simulink library "AERO_lib"  (R2015a)
settings: Solver=ode45  StartTime=0.0  StopTime=10.0  RelTol=1e-3
values from neighbouring files (symbols this model uses):
  VAF = {}    [setup_aero.m]
libraries: simulink x8
settings Model: Creator=Andrew  LastModifiedBy=Andrew

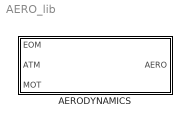
== system AERO_lib ==
  AERODYNAMICS : Subsystem

== system AERO_lib/AERODYNAMICS ==
  EOM : Inport
  ATM : Inport  Port=2
  MOT : Inport  Port=3
  AERODYNAMIC PROPERTIES : Subsystem
  Bus Creator : BusCreator  Inputs=6
  Bus Selector : BusSelector  OutputSignals=SONIC_VEL,TEMP,RHO
  Bus Selector1 : BusSelector  OutputSignals=signal1,signal2
  Bus Selector2 : BusSelector  OutputSignals=signal1,signal2
  AERO : Outport
  wires:
  Bus Selector2/2 -> AERODYNAMIC PROPERTIES/8(MOTOR DIAMETER)  "<signal2>"
  Bus Selector2/1 -> AERODYNAMIC PROPERTIES/7(THRUST ACTIVE)  "<signal1>"
  Bus Selector/3 -> AERODYNAMIC PROPERTIES/6(RHO)  "<RHO>"
  Bus Selector/2 -> AERODYNAMIC PROPERTIES/5(TEMP)  "<TEMP>"
  Bus Selector/1 -> AERODYNAMIC PROPERTIES/4(a (m/s))  "<SONIC_VEL>"
  AERODYNAMIC PROPERTIES/1(X_CP_TOT) -> Bus Creator/1  "X_CP"
  AERODYNAMIC PROPERTIES/2(X_CP_FIN) -> Bus Creator/2  "FIN_CP"
  AERODYNAMIC PROPERTIES/3(Reynolds Number) -> Bus Creator/3  "Re"
  AERODYNAMIC PROPERTIES/4(Cm_Damp) -> Bus Creator/4  "CM_DAMP"
  AERODYNAMIC PROPERTIES/5(CD_TOTAL) -> Bus Creator/5  "CD_TOT"
  AERODYNAMIC PROPERTIES/6(CD_ALL) -> Bus Creator/6  "CD_ALL"
  Bus Creator/1 -> AERO/1
  ATM/1 -> Bus Selector/1
  EOM/1 -> Bus Selector1/1
  MOT/1 -> Bus Selector2/1

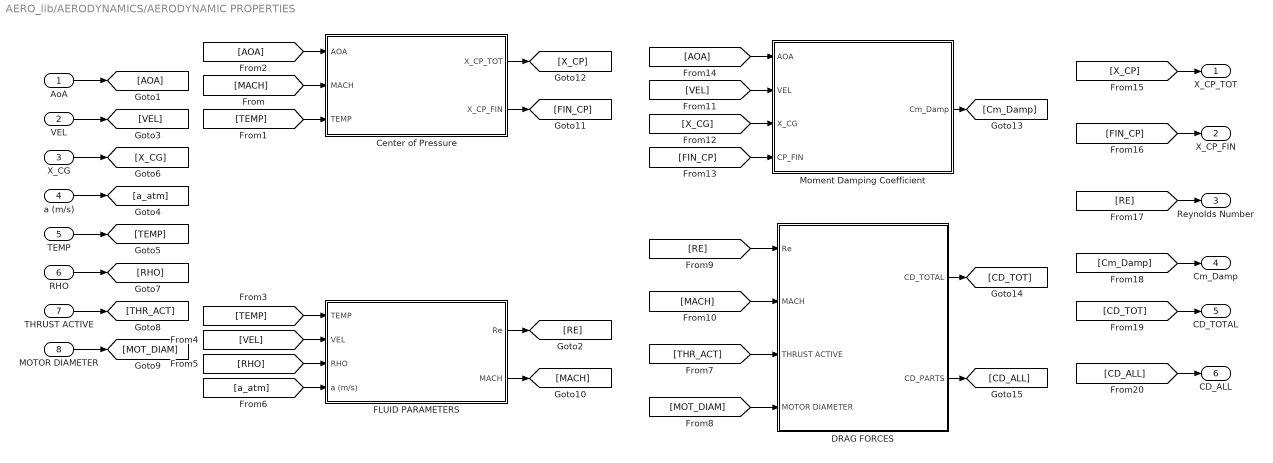
== system AERO_lib/AERODYNAMICS/AERODYNAMIC PROPERTIES ==
  AoA : Inport
  VEL : Inport  Port=2
  X_CG : Inport  Port=3
  a (m/s) : Inport  Port=4
  TEMP : Inport  Port=5
  RHO : Inport  Port=6
  THRUST ACTIVE : Inport  Port=7
  MOTOR DIAMETER : Inport  Port=8
  Center of Pressure : Subsystem
  DRAG FORCES : Subsystem
  FLUID PARAMETERS : Subsystem
  Moment Damping Coefficient : Subsystem
  X_CP_TOT : Outport
  X_CP_FIN : Outport  Port=2
  Reynolds Number : Outport  Port=3
  Cm_Damp : Outport  Port=4
  CD_TOTAL : Outport  Port=5
  CD_ALL : Outport  Port=6
  wires:
  a (m/s)/1 -> [a_atm]
  AoA/1 -> [AOA]
  VEL/1 -> [VEL]
  TEMP/1 -> [TEMP]
  X_CG/1 -> [X_CG]
  RHO/1 -> [RHO]
  THRUST ACTIVE/1 -> [THR_ACT]
  MOTOR DIAMETER/1 -> [MOT_DIAM]
  [MACH] -> Center of Pressure/2(MACH)
  [TEMP] -> Center of Pressure/3(TEMP)
  [AOA] -> Center of Pressure/1(AOA)
  [TEMP] -> FLUID PARAMETERS/1(TEMP)
  [RHO] -> FLUID PARAMETERS/3(RHO)
  [a_atm] -> FLUID PARAMETERS/4(a (m/s))
  [VEL] -> FLUID PARAMETERS/2(VEL)
  [THR_ACT] -> DRAG FORCES/3(THRUST ACTIVE)
  [MOT_DIAM] -> DRAG FORCES/4(MOTOR DIAMETER)
  [MACH] -> DRAG FORCES/2(MACH)
  [RE] -> DRAG FORCES/1(Re)
  FLUID PARAMETERS/1(Re) -> [RE]
  FLUID PARAMETERS/2(MACH) -> [MACH]
  Center of Pressure/1(X_CP_TOT) -> [X_CP]
  Center of Pressure/2(X_CP_FIN) -> [FIN_CP]
  [AOA] -> Moment Damping Coefficient/1(AOA)
  [VEL] -> Moment Damping Coefficient/2(VEL)
  [X_CG] -> Moment Damping Coefficient/3(X_CG)
  [FIN_CP] -> Moment Damping Coefficient/4(CP_FIN)
  DRAG FORCES/1(CD_TOTAL) -> [CD_TOT]
  DRAG FORCES/2(CD_PARTS) -> [CD_ALL]
  Moment Damping Coefficient/1(Cm_Damp) -> [Cm_Damp]
  [X_CP] -> X_CP_TOT/1
  [FIN_CP] -> X_CP_FIN/1
  [RE] -> Reynolds Number/1
  [Cm_Damp] -> Cm_Damp/1
  [CD_TOT] -> CD_TOTAL/1
  [CD_ALL] -> CD_ALL/1

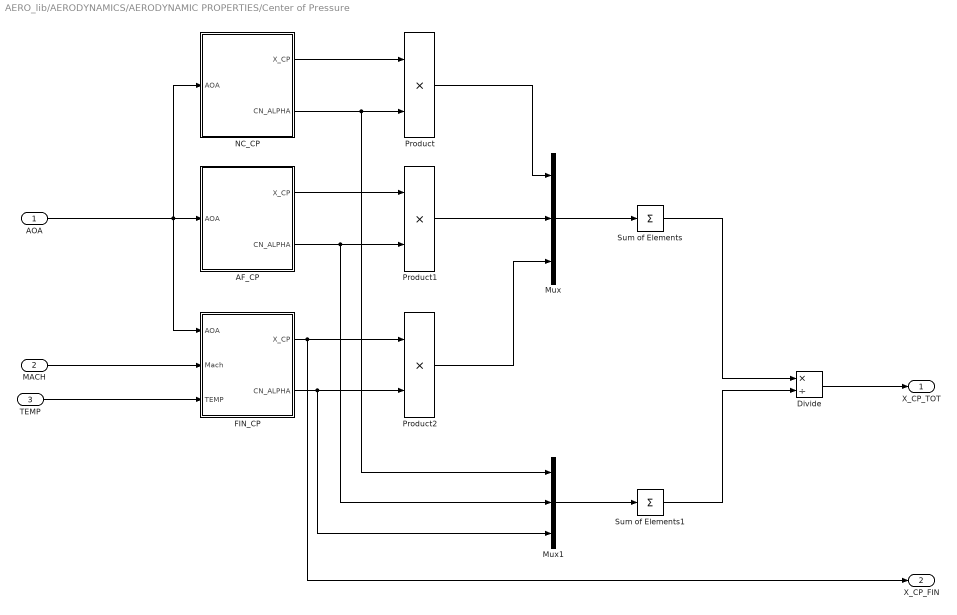
== system AERO_lib/AERODYNAMICS/AERODYNAMIC PROPERTIES/Center of Pressure ==
  AOA : Inport
  MACH : Inport  Port=2
  TEMP : Inport  Port=3
  AF_CP : Subsystem
  Divide : Product  Inputs=*/
  FIN_CP : Subsystem
  Mux : Mux  Inputs=3
  Mux1 : Mux  Inputs=3
  NC_CP : Subsystem
  Product : Product
  Product1 : Product
  Product2 : Product
  Sum of Elements : Sum  Inputs=+
  Sum of Elements1 : Sum  Inputs=+
  X_CP_TOT : Outport
  X_CP_FIN : Outport  Port=2
  wires:
  AOA/1 -> FIN_CP/1(AOA), NC_CP/1(AOA), AF_CP/1(AOA)
  MACH/1 -> FIN_CP/2(Mach)
  NC_CP/1(X_CP) -> Product/1
  AF_CP/2(CN_ALPHA) -> Mux1/2, Product1/2
  Product1/1 -> Mux/2
  Divide/1 -> X_CP_TOT/1
  Sum of Elements/1 -> Divide/1
  Product/1 -> Mux/1
  Mux1/1 -> Sum of Elements1/1
  AF_CP/1(X_CP) -> Product1/1
  NC_CP/2(CN_ALPHA) -> Mux1/1, Product/2
  Mux/1 -> Sum of Elements/1
  Sum of Elements1/1 -> Divide/2
  FIN_CP/1(X_CP) -> X_CP_FIN/1, Product2/1
  Product2/1 -> Mux/3
  FIN_CP/2(CN_ALPHA) -> Product2/2, Mux1/3
  TEMP/1 -> FIN_CP/3(TEMP)

== system AERO_lib/AERODYNAMICS/AERODYNAMIC PROPERTIES/DRAG FORCES ==
  Re : Inport
  MACH : Inport  Port=2
  THRUST ACTIVE : Inport  Port=3
  MOTOR DIAMETER : Inport  Port=4
  Add : Sum
  Body Drag : Subsystem
  Mux : Mux  Inputs=2
  Skin Friction Drag : Subsystem
  CD_TOTAL : Outport
  CD_PARTS : Outport  Port=2
  wires:
  MACH/1 -> Body Drag/1(MACH), Skin Friction Drag/2(MACH)
  Re/1 -> Skin Friction Drag/1(Re)
  MOTOR DIAMETER/1 -> Body Drag/3(MOTOR DIAMETER)
  THRUST ACTIVE/1 -> Body Drag/2(THRUST ACTIVE)
  Body Drag/1(CD_BODY) -> Add/2
  Skin Friction Drag/1(Cd_Fric) -> Mux/2, Add/1
  Add/1 -> CD_TOTAL/1
  Body Drag/2(CD_PARTS) -> Mux/1
  Mux/1 -> CD_PARTS/1

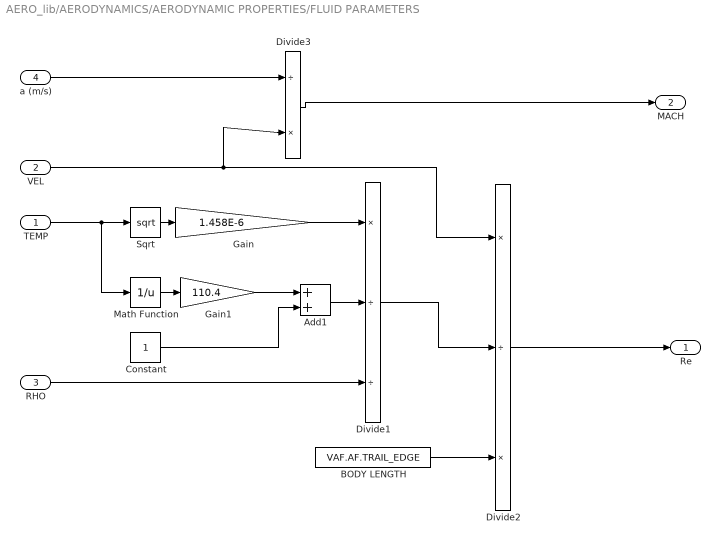
== system AERO_lib/AERODYNAMICS/AERODYNAMIC PROPERTIES/FLUID PARAMETERS ==
  TEMP : Inport
  VEL : Inport  Port=2
  RHO : Inport  Port=3
  a (m/s) : Inport  Port=4
  Add1 : Sum
  BODY LENGTH : FromWorkspace  VariableName=VAF.AF.TRAIL_EDGE  SampleTime=0
  Constant : Constant
  Divide1 : Product  Inputs=*//
  Divide2 : Product  Inputs=*/*
  Divide3 : Product  Inputs=/*
  Gain : Gain  Gain=1.458E-6
  Gain1 : Gain  Gain=110.4
  Math Function : Math  Operator=reciprocal  SaturateOnIntegerOverflow=on
  Sqrt : Sqrt  SaturateOnIntegerOverflow=on
  Re : Outport
  MACH : Outport  Port=2
  wires:
  Constant/1 -> Add1/2
  Math Function/1 -> Gain1/1
  Gain1/1 -> Add1/1
  RHO/1 -> Divide1/3
  Add1/1 -> Divide1/2
  BODY LENGTH/1 -> Divide2/3
  Divide1/1 -> Divide2/2
  Sqrt/1 -> Gain/1
  Gain/1 -> Divide1/1
  Divide2/1 -> Re/1
  VEL/1 -> Divide3/2, Divide2/1
  TEMP/1 -> Math Function/1, Sqrt/1
  a (m/s)/1 -> Divide3/1
  Divide3/1 -> MACH/1

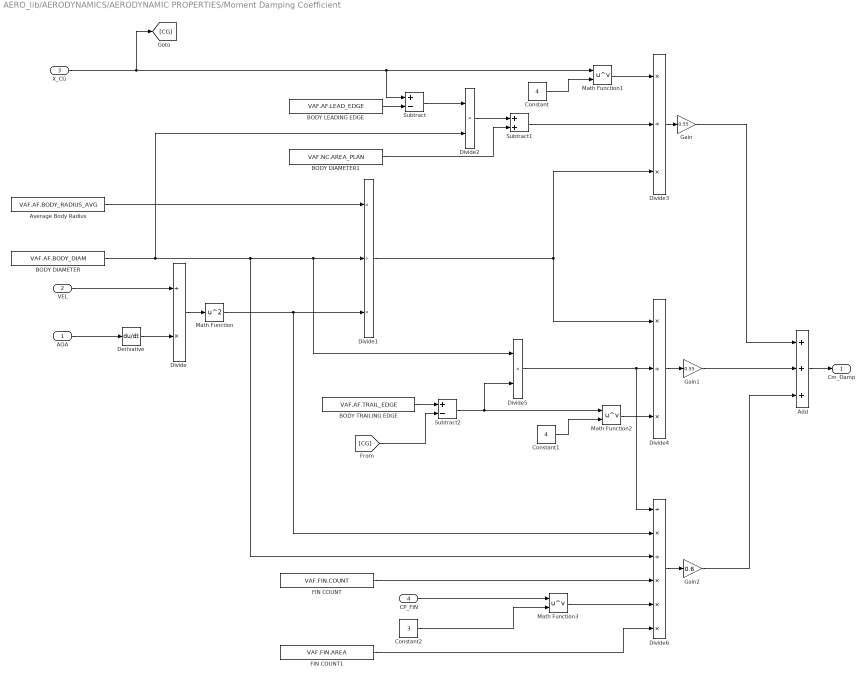
== system AERO_lib/AERODYNAMICS/AERODYNAMIC PROPERTIES/Moment Damping Coefficient ==
  AOA : Inport
  VEL : Inport  Port=2
  X_CG : Inport  Port=3
  CP_FIN : Inport  Port=4
  Add : Sum  Inputs=+++
  Average Body Radius : FromWorkspace  VariableName=VAF.AF.BODY_RADIUS_AVG  SampleTime=0
  BODY DIAMETER : FromWorkspace  VariableName=VAF.AF.BODY_DIAM  SampleTime=0
  BODY DIAMETER1 : FromWorkspace  VariableName=VAF.NC.AREA_PLAN  SampleTime=0
  BODY LEADING EDGE : FromWorkspace  VariableName=VAF.AF.LEAD_EDGE  SampleTime=0
  BODY TRAILING EDGE : FromWorkspace  VariableName=VAF.AF.TRAIL_EDGE  SampleTime=0
  Constant : Constant  Value=4
  Constant1 : Constant  Value=4
  Constant2 : Constant  Value=3
  Derivative : Derivative
  Divide : Product  Inputs=/*
  Divide1 : Product  Inputs=*/*
  Divide2 : Product  Inputs=**
  Divide3 : Product  Inputs=*/*
  Divide4 : Product  Inputs=*/*
  Divide5 : Product  Inputs=**
  Divide6 : Product  Inputs=/*/***
  FIN COUNT : FromWorkspace  VariableName=VAF.FIN.COUNT  SampleTime=0
  FIN COUNT1 : FromWorkspace  VariableName=VAF.FIN.AREA  SampleTime=0
  Gain : Gain  Gain=0.55
  Gain1 : Gain  Gain=0.55
  Gain2 : Gain  Gain=0.6
  Math Function : Math  Operator=square  SaturateOnIntegerOverflow=on
  Math Function1 : Math  Operator=pow  SaturateOnIntegerOverflow=on
  Math Function2 : Math  Operator=pow  SaturateOnIntegerOverflow=on
  Math Function3 : Math  Operator=pow  SaturateOnIntegerOverflow=on
  Subtract : Sum  Inputs=+-
  Subtract1 : Sum
  Subtract2 : Sum  Inputs=+-
  Cm_Damp : Outport
  wires:
  AOA/1 -> Derivative/1
  Derivative/1 -> Divide/2
  VEL/1 -> Divide/1
  Divide/1 -> Math Function/1
  Math Function/1 -> Divide6/2, Divide1/3
  BODY LEADING EDGE/1 -> Subtract/2
  Divide2/1 -> Subtract1/1
  Constant/1 -> Math Function1/2
  Subtract/1 -> Divide2/1
  Subtract1/1 -> Divide3/2
  BODY DIAMETER1/1 -> Subtract1/2
  Average Body Radius/1 -> Divide1/1
  BODY DIAMETER/1 -> Divide6/3, Divide5/1, Divide1/2, Divide2/2
  X_CG/1 -> [CG], Subtract/1, Math Function1/1
  Math Function1/1 -> Divide3/1
  Divide1/1 -> Divide4/1, Divide3/3
  Divide3/1 -> Gain/1
  BODY TRAILING EDGE/1 -> Subtract2/1
  [CG] -> Subtract2/2
  Divide5/1 -> Divide6/1, Divide4/2
  Subtract2/1 -> Math Function2/1, Divide5/2
  Math Function2/1 -> Divide4/3
  Constant1/1 -> Math Function2/2
  Divide4/1 -> Gain1/1
  CP_FIN/1 -> Math Function3/1
  Constant2/1 -> Math Function3/2
  Math Function3/1 -> Divide6/5
  FIN COUNT/1 -> Divide6/4
  FIN COUNT1/1 -> Divide6/6
  Divide6/1 -> Gain2/1
  Gain1/1 -> Add/2
  Gain2/1 -> Add/3
  Gain/1 -> Add/1
  Add/1 -> Cm_Damp/1

== system AERO_lib/AERODYNAMICS/AERODYNAMIC PROPERTIES/Center of Pressure/AF_CP ==
  AOA : Inport
  Add : Sum
  Compare To Zero : simulink/Logic and Bit Operations/Compare To Zero  relop=~=  OutDataTypeStr=boolean
  Constant : Constant
  Divide : Product  Inputs=*/*
  Divide1 : Product  Inputs=*/
  LEADING EDGE AREA : FromWorkspace  VariableName=VAF.AF.LEAD_EDGE_AREA
  LEADING EDGE OFFSET : FromWorkspace  VariableName=VAF.AC.LEAD_EDGE
  NOSECONE CP : FromWorkspace  VariableName=VAF.AF.X_CP
  REFERENCE AREA : FromWorkspace  VariableName=VAF.AF.AREA_REF
  Subtract : Sum  Inputs=+-
  Switch : Switch  Criteria=u2 ~= 0
  TRAILING EDGE AREA : FromWorkspace  VariableName=VAF.AF.TRAIL_EDGE_AREA
  Trigonometric Function : Trigonometry  OutputSignalType=real
  X_CP : Outport
  CN_ALPHA : Outport  Port=2
  wires:
  Divide1/1 -> Switch/1
  Trigonometric Function/1 -> Divide1/1
  LEADING EDGE AREA/1 -> Subtract/1
  TRAILING EDGE AREA/1 -> Subtract/2
  Subtract/1 -> Divide/1
  AOA/1 -> Compare To Zero/1, Divide1/2, Trigonometric Function/1
  Constant/1 -> Switch/3
  Compare To Zero/1 -> Switch/2
  Switch/1 -> Divide/3
  Divide/1 -> CN_ALPHA/1
  REFERENCE AREA/1 -> Divide/2
  Add/1 -> X_CP/1
  LEADING EDGE OFFSET/1 -> Add/2
  NOSECONE CP/1 -> Add/1

== system AERO_lib/AERODYNAMICS/AERODYNAMIC PROPERTIES/Center of Pressure/FIN_CP ==
  AOA : Inport
  Mach : Inport  Port=2
  TEMP : Inport  Port=3
  FIN CP : Subsystem
  SINGLE FIN CN_ALPHA : Subsystem
  TOTAL FIN CN_ALPHA : Subsystem
  X_CP : Outport
  CN_ALPHA : Outport  Port=2
  wires:
  Mach/1 -> SINGLE FIN CN_ALPHA/1(MACH), FIN CP/1(MACH)
  FIN CP/1(X_CP) -> X_CP/1
  AOA/1 -> SINGLE FIN CN_ALPHA/2(AOA)
  TEMP/1 -> SINGLE FIN CN_ALPHA/3(TEMP)
  SINGLE FIN CN_ALPHA/1(CN_ALPHA) -> TOTAL FIN CN_ALPHA/1(CN_ALPHA_1)
  TOTAL FIN CN_ALPHA/1(CN_ALPHA_FINAL) -> CN_ALPHA/1

== system AERO_lib/AERODYNAMICS/AERODYNAMIC PROPERTIES/Center of Pressure/NC_CP ==
  AOA : Inport
  Add : Sum
  Compare To Zero : simulink/Logic and Bit Operations/Compare To Zero  relop=~=  OutDataTypeStr=boolean
  Constant : Constant
  Divide : Product  Inputs=*/*
  Divide1 : Product  Inputs=*/
  LEADING EDGE AREA : FromWorkspace  VariableName=VAF.NC.LEAD_EDGE_AREA
  LEADING EDGE OFFSET : FromWorkspace  VariableName=VAF.NC.LEAD_EDGE
  NOSECONE CP : FromWorkspace  VariableName=VAF.NC.X_CP
  REFERENCE AREA : FromWorkspace  VariableName=VAF.NC.AREA_REF
  Subtract : Sum  Inputs=+-
  Switch : Switch  Criteria=u2 ~= 0
  TRAILING EDGE AREA : FromWorkspace  VariableName=VAF.NC.TRAIL_EDGE_AREA
  Trigonometric Function : Trigonometry  OutputSignalType=real
  X_CP : Outport
  CN_ALPHA : Outport  Port=2
  wires:
  NOSECONE CP/1 -> Add/1
  LEADING EDGE OFFSET/1 -> Add/2
  Add/1 -> X_CP/1
  Divide/1 -> CN_ALPHA/1
  REFERENCE AREA/1 -> Divide/2
  Switch/1 -> Divide/3
  Compare To Zero/1 -> Switch/2
  Constant/1 -> Switch/3
  AOA/1 -> Trigonometric Function/1, Divide1/2, Compare To Zero/1
  Subtract/1 -> Divide/1
  TRAILING EDGE AREA/1 -> Subtract/2
  LEADING EDGE AREA/1 -> Subtract/1
  Trigonometric Function/1 -> Divide1/1
  Divide1/1 -> Switch/1

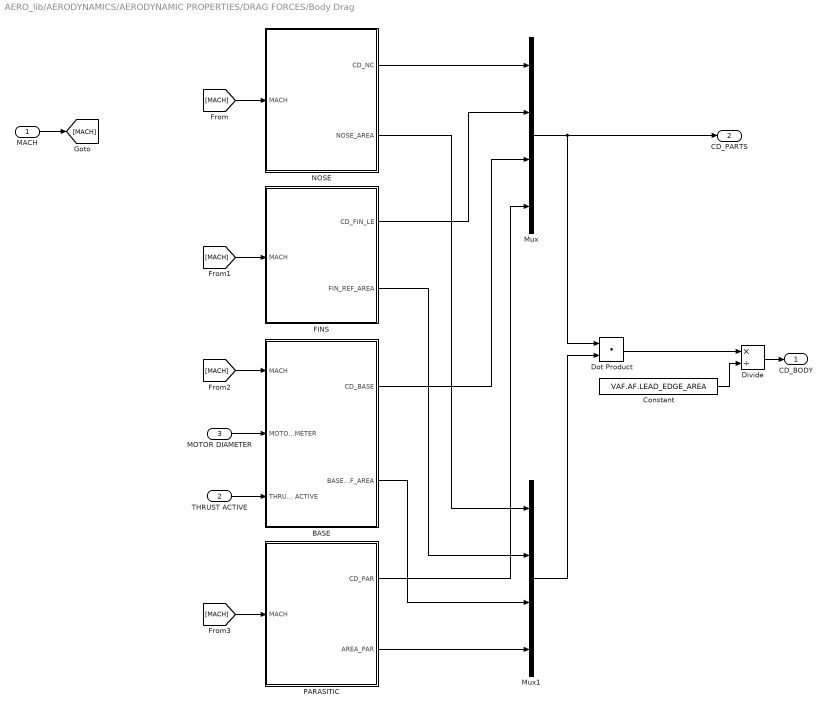
== system AERO_lib/AERODYNAMICS/AERODYNAMIC PROPERTIES/DRAG FORCES/Body Drag ==
  MACH : Inport
  THRUST ACTIVE : Inport  Port=2
  MOTOR DIAMETER : Inport  Port=3
  BASE : Subsystem
  Constant : Constant  Value=VAF.AF.LEAD_EDGE_AREA
  Divide : Product  Inputs=*/
  Dot Product : DotProduct  InputSameDT=on  OutDataTypeStr=Inherit: Inherit via internal rule
  FINS : Subsystem
  Mux : Mux
  Mux1 : Mux
  NOSE : Subsystem
  PARASITIC : Subsystem
  CD_BODY : Outport
  CD_PARTS : Outport  Port=2
  wires:
  MACH/1 -> [MACH]
  [MACH] -> NOSE/1(MACH)
  [MACH] -> FINS/1(MACH)
  [MACH] -> BASE/1(MACH)
  MOTOR DIAMETER/1 -> BASE/2(MOTOR DIAMETER)
  THRUST ACTIVE/1 -> BASE/3(THRUST ACTIVE)
  [MACH] -> PARASITIC/1(MACH)
  NOSE/1(CD_NC) -> Mux/1
  FINS/1(CD_FIN_LE) -> Mux/2
  BASE/1(CD_BASE) -> Mux/3
  PARASITIC/1(CD_PAR) -> Mux/4
  PARASITIC/2(AREA_PAR) -> Mux1/4
  BASE/2(BASE_REF_AREA) -> Mux1/3
  FINS/2(FIN_REF_AREA) -> Mux1/2
  NOSE/2(NOSE_AREA) -> Mux1/1
  Mux1/1 -> Dot Product/2
  Mux/1 -> Dot Product/1, CD_PARTS/1
  Dot Product/1 -> Divide/1
  Divide/1 -> CD_BODY/1
  Constant/1 -> Divide/2

== system AERO_lib/AERODYNAMICS/AERODYNAMIC PROPERTIES/DRAG FORCES/Skin Friction Drag ==
  Re : Inport
  MACH : Inport  Port=2
  Compressibility Corrections : Subsystem
  Friction Drag Coefficient : Subsystem
  RE-BASED FRIC. COEFF : Subsystem
  Cd_Fric : Outport
  wires:
  Re/1 -> RE-BASED FRIC. COEFF/1(RE)
  RE-BASED FRIC. COEFF/1(CF_Skin) -> Compressibility Corrections/1(RE)
  MACH/1 -> Compressibility Corrections/2(CF_skin)
  Compressibility Corrections/1(CF_Skin) -> Friction Drag Coefficient/1(CF_Skin)
  Friction Drag Coefficient/1(Cd_Fric) -> Cd_Fric/1

== system AERO_lib/AERODYNAMICS/AERODYNAMIC PROPERTIES/Center of Pressure/FIN_CP/FIN CP ==
  MACH : Inport
  CP_SUPERSONIC : Subsystem
  Compare To Constant : simulink/Logic and Bit Operations/Compare To Constant  relop=>  const=0.5  OutDataTypeStr=boolean
  Compare To Constant1 : simulink/Logic and Bit Operations/Compare To Constant  relop=>=  const=2.0  OutDataTypeStr=boolean
  Gain : Gain  Gain=VAF.FIN.MAC
  Polynomial : Polyval  Coefs=VAF.FIN.MACH_CP_COEFFS
  Switch1 : Switch  Criteria=u2 ~= 0
  Switch2 : Switch  Criteria=u2 ~= 0
  XF_SUBSONIC : FromWorkspace  VariableName=VAF.FIN.X_F_SUBSONIC
  X_CP : Outport
  wires:
  Switch1/1 -> X_CP/1
  MACH/1 -> Polynomial/1, Compare To Constant/1, CP_SUPERSONIC/1(Mach), Compare To Constant1/1
  CP_SUPERSONIC/1(X_F_SUPERSONIC) -> Switch2/1
  Switch2/1 -> Switch1/1
  Compare To Constant/1 -> Switch1/2
  Compare To Constant1/1 -> Switch2/2
  XF_SUBSONIC/1 -> Switch1/3
  Polynomial/1 -> Gain/1
  Gain/1 -> Switch2/3

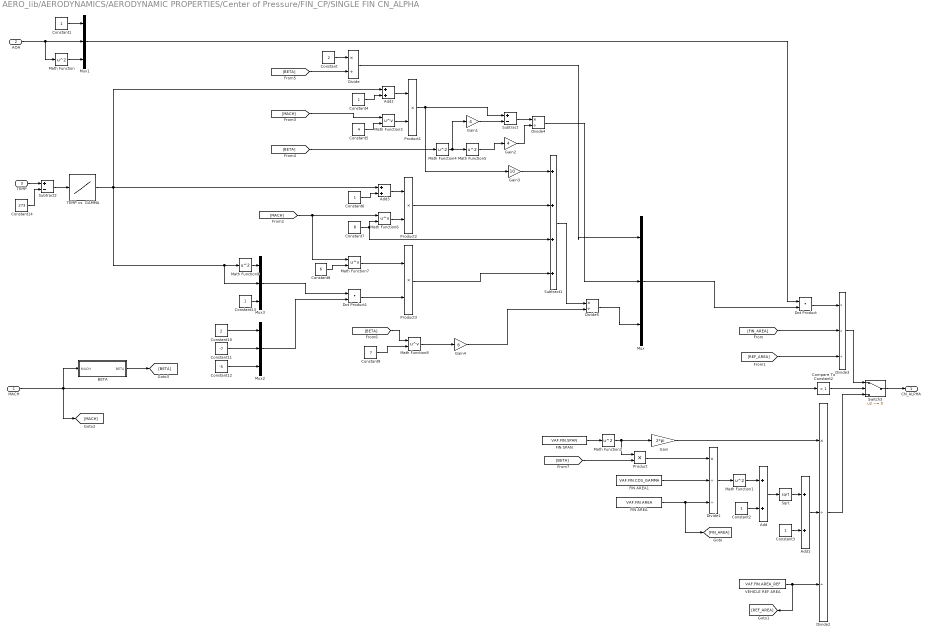
== system AERO_lib/AERODYNAMICS/AERODYNAMIC PROPERTIES/Center of Pressure/FIN_CP/SINGLE FIN CN_ALPHA ==
  MACH : Inport
  AOA : Inport  Port=2
  TEMP : Inport  Port=3
  Add{,1..3} (4 alike) : Sum
  BETA : Subsystem
  Compare To Constant2 : simulink/Logic and Bit Operations/Compare To Constant  relop=>  const=1  OutDataTypeStr=boolean
  Constant : Constant  Value=2
  Constant{1..4,6,13} (6 alike) : Constant
  Constant10 : Constant  Value=2
  Constant11 : Constant  Value=-7
  Constant12 : Constant  Value=-5
  Constant14 : Constant  Value=273
  Constant5 : Constant  Value=4
  Constant7 : Constant  Value=8
  Constant8 : Constant  Value=6
  Constant9 : Constant  Value=7
  Divide : Product  Inputs=*/
  Divide1 : Product  Inputs=*//
  Divide2 : Product  Inputs=*//
  Divide3 : Product  Inputs=**/
  Divide4 : Product  Inputs=*/
  Divide5 : Product  Inputs=*/
  Dot Product : DotProduct  InputSameDT=on  OutDataTypeStr=Inherit: Inherit via internal rule
  Dot Product1 : DotProduct  InputSameDT=on  OutDataTypeStr=Inherit: Inherit via internal rule
  FIN AREA : FromWorkspace  VariableName=VAF.FIN.AREA  SampleTime=0
  FIN AREA1 : FromWorkspace  VariableName=VAF.FIN.COS_GAMMA  SampleTime=0
  FIN SPAN : FromWorkspace  VariableName=VAF.FIN.SPAN  SampleTime=0
  Gain : Gain  Gain=2*pi
  Gain1 : Gain  Gain=4
  Gain2 : Gain  Gain=4
  Gain3 : Gain  Gain=10
  Gain4 : Gain  Gain=6
  Math Function{,1..2,4..5,9} (6 alike) : Math  Operator=square  SaturateOnIntegerOverflow=on
  Math Function{3,6..8} (4 alike) : Math  Operator=pow  SaturateOnIntegerOverflow=on
  Mux{,1..3} (4 alike) : Mux  Inputs=3
  Product{,1..3} (4 alike) : Product
  Sqrt : Sqrt  SaturateOnIntegerOverflow=on
  Subtract : Sum  Inputs=+-
  Subtract1 : Sum  Inputs=++++
  Subtract2 : Sum  Inputs=+-
  Switch3 : Switch  Criteria=u2 ~= 0
  TEMP vs. GAMMA : Lookup_n-D  NumberOfTableDimensions=1  BreakpointsForDimension1=VAF.GAS.GAMMA_VS_TEMP(:,1)  Table=VAF.GAS.GAMMA_VS_TEMP(:,2)  InternalRulePriority=Speed  RndMeth=Simplest  InputSameDT=on
  VEHICLE REF AREA : FromWorkspace  VariableName=VAF.FIN.AREA_REF  SampleTime=0
  CN_ALPHA : Outport
  wires:
  Mux1/1 -> Dot Product/1
  Mux/1 -> Dot Product/2
  Mux2/1 -> Dot Product1/2
  Divide/1 -> Mux/1
  FIN AREA/1 -> [FIN_AREA], Divide1/3
  Product/1 -> Divide1/1
  FIN AREA1/1 -> Divide1/2
  Math Function1/1 -> Add/1
  Divide1/1 -> Math Function1/1
  Constant/1 -> Divide/1
  Math Function2/1 -> Gain/1, Product/1
  FIN SPAN/1 -> Math Function2/1
  Gain3/1 -> Subtract1/1
  Math Function5/1 -> Gain2/1
  Gain/1 -> Divide2/1
  AOA/1 -> Math Function/1, Mux1/2
  Add/1 -> Sqrt/1
  Constant10/1 -> Mux2/1
  Mux3/1 -> Dot Product1/1
  Constant13/1 -> Mux3/3
  Switch3/1 -> CN_ALPHA/1
  Compare To Constant2/1 -> Switch3/2
  Gain2/1 -> Divide4/2
  Math Function4/1 -> Gain1/1, Math Function5/1
  Divide5/1 -> Mux/3
  Constant1/1 -> Mux1/1
  Constant12/1 -> Mux2/3
  Constant9/1 -> Math Function8/2
  Constant4/1 -> Add2/2
  TEMP vs. GAMMA/1 -> Add3/1, Add2/1, Mux3/2, Math Function9/1
  VEHICLE REF AREA/1 -> [REF_AREA], Divide2/3
  Add2/1 -> Product1/1
  Math Function3/1 -> Product1/2
  Math Function6/1 -> Product2/2
  Product2/1 -> Subtract1/2
  Constant7/1 -> Subtract1/3, Math Function6/2
  Add3/1 -> Product2/1
  Constant6/1 -> Add3/2
  Dot Product/1 -> Divide3/1
  [FIN_AREA] -> Divide3/2
  [REF_AREA] -> Divide3/3
  Divide3/1 -> Switch3/1
  Math Function9/1 -> Mux3/1
  Add1/1 -> Divide2/2
  Sqrt/1 -> Add1/1
  Constant3/1 -> Add1/2
  Divide2/1 -> Switch3/3
  Gain4/1 -> Divide5/2
  Math Function/1 -> Mux1/3
  Constant2/1 -> Add/2
  Product3/1 -> Subtract1/4
  Math Function7/1 -> Product3/1
  Constant8/1 -> Math Function7/2
  Subtract1/1 -> Divide5/1
  Dot Product1/1 -> Product3/2
  Constant11/1 -> Mux2/2
  Constant5/1 -> Math Function3/2
  Gain1/1 -> Subtract/2
  Product1/1 -> Gain3/1, Subtract/1
  Subtract/1 -> Divide4/1
  Divide4/1 -> Mux/2
  Math Function8/1 -> Gain4/1
  BETA/1(BETA) -> [BETA]
  MACH/1 -> BETA/1(MACH), Compare To Constant2/1, [MACH]
  [MACH] -> Math Function7/1, Math Function6/1
  [MACH] -> Math Function3/1
  [BETA] -> Math Function4/1
  [BETA] -> Divide/2
  [BETA] -> Math Function8/1
  [BETA] -> Product/2
  Subtract2/1 -> TEMP vs. GAMMA/1
  TEMP/1 -> Subtract2/1
  Constant14/1 -> Subtract2/2

== system AERO_lib/AERODYNAMICS/AERODYNAMIC PROPERTIES/Center of Pressure/FIN_CP/TOTAL FIN CN_ALPHA ==
  CN_ALPHA_1 : Inport
  1-D Lookup Table : Lookup_n-D  NumberOfTableDimensions=1  BreakpointsForDimension1=VAF.FIN.INTERFERE_CORR(:,1)'  Table=VAF.FIN.INTERFERE_CORR(:,2)'  InternalRulePriority=Speed  RndMeth=Simplest  InputSameDT=on
  Add : Sum
  Constant : Constant
  Divide : Product  Inputs=*/
  FIN BODY DIAMETER : FromWorkspace  VariableName=VAF.FIN.BODY_DIAM  SampleTime=0
  FIN COUNT : FromWorkspace  VariableName=VAF.FIN.COUNT  SampleTime=0
  FIN DIHEDRAL ANGLE : FromWorkspace  VariableName=VAF.FIN.LAMBDA_VEC  SampleTime=0
  FIN SPAN : FromWorkspace  VariableName=VAF.FIN.SPAN  SampleTime=0
  Gain : Gain  Gain=0.5
  Math Function : Math  Operator=square  SaturateOnIntegerOverflow=on
  Product : Product  Inputs=4
  Subtract : Sum
  Sum of Elements : Sum  Inputs=+
  Trigonometric Function : Trigonometry
  CN_ALPHA_FINAL : Outport
  wires:
  FIN DIHEDRAL ANGLE/1 -> Trigonometric Function/1
  Trigonometric Function/1 -> Math Function/1
  Math Function/1 -> Sum of Elements/1
  CN_ALPHA_1/1 -> Product/1
  Sum of Elements/1 -> Product/2
  Product/1 -> CN_ALPHA_FINAL/1
  FIN COUNT/1 -> 1-D Lookup Table/1
  1-D Lookup Table/1 -> Product/3
  Add/1 -> Product/4
  Constant/1 -> Add/1
  FIN BODY DIAMETER/1 -> Gain/1
  Divide/1 -> Add/2
  FIN SPAN/1 -> Subtract/2
  Subtract/1 -> Divide/2
  Gain/1 -> Subtract/1, Divide/1

== system AERO_lib/AERODYNAMICS/AERODYNAMIC PROPERTIES/DRAG FORCES/Body Drag/BASE ==
  MACH : Inport
  MOTOR DIAMETER : Inport  Port=2
  THRUST ACTIVE : Inport  Port=3
  Add2 : Sum
  Constant1 : Constant  Value=VAF.AF.TRAIL_EDGE_AREA
  Gain : Gain  Gain=pi
  If1 : If  IfExpression=u1<1
  Math Function : Math  Operator=square  SaturateOnIntegerOverflow=on
  Product1 : Product
  Subsonic : Subsystem  TreatAsAtomicUnit=on
  Subtract : Sum  Inputs=+-
  Supersonic : Subsystem  TreatAsAtomicUnit=on
  CD_BASE : Outport
  BASE_REF_AREA : Outport  Port=2
  wires:
  Add2/1 -> CD_BASE/1
  Subtract/1 -> BASE_REF_AREA/1
  Constant1/1 -> Subtract/1
  Product1/1 -> Math Function/1
  THRUST ACTIVE/1 -> Product1/2
  MOTOR DIAMETER/1 -> Product1/1
  Gain/1 -> Subtract/2
  Math Function/1 -> Gain/1
  If1/2 -> Supersonic/Action
  If1/1 -> Subsonic/Action
  Subsonic/1(CD_BASE) -> Add2/2
  Supersonic/1(CD_BASE) -> Add2/1
  MACH/1 -> Subsonic/1(MACH), Supersonic/1(MACH), If1/1

== system AERO_lib/AERODYNAMICS/AERODYNAMIC PROPERTIES/DRAG FORCES/Body Drag/FINS ==
  MACH : Inport
  Add : Sum
  Constant : Constant  Value=VAF.FIN.AREA_REF_DRAG
  Leading Edge : Subsystem
  Trailing Edge : Subsystem
  CD_FIN_LE : Outport
  FIN_REF_AREA : Outport  Port=2
  wires:
  Constant/1 -> FIN_REF_AREA/1
  Add/1 -> CD_FIN_LE/1
  Leading Edge/1(CD_FIN_LE) -> Add/1
  Trailing Edge/1(CD_FIN_LE) -> Add/2
  MACH/1 -> Trailing Edge/1(MACH), Leading Edge/1(MACH)

== system AERO_lib/AERODYNAMICS/AERODYNAMIC PROPERTIES/DRAG FORCES/Body Drag/NOSE ==
  MACH : Inport
  Add1 : Sum  Inputs=++++
  CONE CORRECTION FACTOR : Gain  Gain=VAF.NC.CONE_CORRECTION
  Constant : Constant  Value=VAF.AF.LEAD_EDGE_AREA
  HIGH SUBSONIC : Subsystem  TreatAsAtomicUnit=on
  If : If  IfExpression=u1 <=0.8  ElseIfExpressions=(u1 > 0.8) & (u1 <= 1.0), (u1 > 1) & (u1 < 1.3)
  LOW SUBSONIC : Subsystem  TreatAsAtomicUnit=on
  SUPERSONIC : Subsystem  TreatAsAtomicUnit=on
  TRANSONIC : Subsystem  TreatAsAtomicUnit=on
  CD_NC : Outport
  NOSE_AREA : Outport  Port=2
  wires:
  CONE CORRECTION FACTOR/1 -> CD_NC/1
  LOW SUBSONIC/1(Out1) -> Add1/1
  HIGH SUBSONIC/1(Cd_NC) -> Add1/4
  TRANSONIC/1(Cd_NC) -> Add1/3
  If/3 -> TRANSONIC/Action
  If/1 -> LOW SUBSONIC/Action
  SUPERSONIC/1(Cd_NC) -> Add1/2
  Add1/1 -> CONE CORRECTION FACTOR/1
  If/2 -> HIGH SUBSONIC/Action
  If/4 -> SUPERSONIC/Action
  MACH/1 -> HIGH SUBSONIC/1(MACH), TRANSONIC/1(MACH), SUPERSONIC/1(MACH), If/1
  Constant/1 -> NOSE_AREA/1

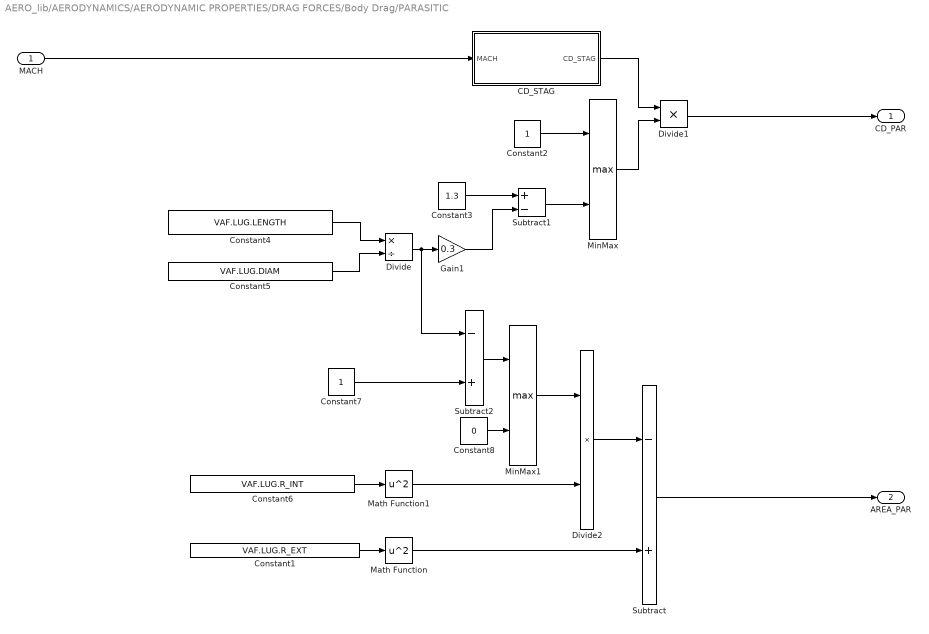
== system AERO_lib/AERODYNAMICS/AERODYNAMIC PROPERTIES/DRAG FORCES/Body Drag/PARASITIC ==
  MACH : Inport
  CD_STAG : Subsystem
  Constant1 : Constant  Value=VAF.LUG.R_EXT
  Constant2 : Constant
  Constant3 : Constant  Value=1.3
  Constant4 : Constant  Value=VAF.LUG.LENGTH
  Constant5 : Constant  Value=VAF.LUG.DIAM
  Constant6 : Constant  Value=VAF.LUG.R_INT
  Constant7 : Constant
  Constant8 : Constant  Value=0
  Divide : Product  Inputs=*/
  Divide1 : Product  Inputs=**
  Divide2 : Product  Inputs=**
  Gain1 : Gain  Gain=0.3
  Math Function : Math  Operator=square  SaturateOnIntegerOverflow=on
  Math Function1 : Math  Operator=square  SaturateOnIntegerOverflow=on
  MinMax : MinMax  Function=max  Inputs=2
  MinMax1 : MinMax  Function=max  Inputs=2
  Subtract : Sum  Inputs=-+
  Subtract1 : Sum  Inputs=+-
  Subtract2 : Sum  Inputs=-+
  CD_PAR : Outport
  AREA_PAR : Outport  Port=2
  wires:
  Divide1/1 -> CD_PAR/1
  Subtract1/1 -> MinMax/2
  Constant3/1 -> Subtract1/1
  Gain1/1 -> Subtract1/2
  Constant2/1 -> MinMax/1
  Divide/1 -> Subtract2/1, Gain1/1
  Constant5/1 -> Divide/2
  Constant4/1 -> Divide/1
  CD_STAG/1(CD_STAG) -> Divide1/1
  MinMax/1 -> Divide1/2
  MACH/1 -> CD_STAG/1(MACH)
  Constant1/1 -> Math Function/1
  Math Function/1 -> Subtract/2
  Constant6/1 -> Math Function1/1
  Constant7/1 -> Subtract2/2
  Subtract2/1 -> MinMax1/1
  Constant8/1 -> MinMax1/2
  MinMax1/1 -> Divide2/1
  Math Function1/1 -> Divide2/2
  Divide2/1 -> Subtract/1
  Subtract/1 -> AREA_PAR/1

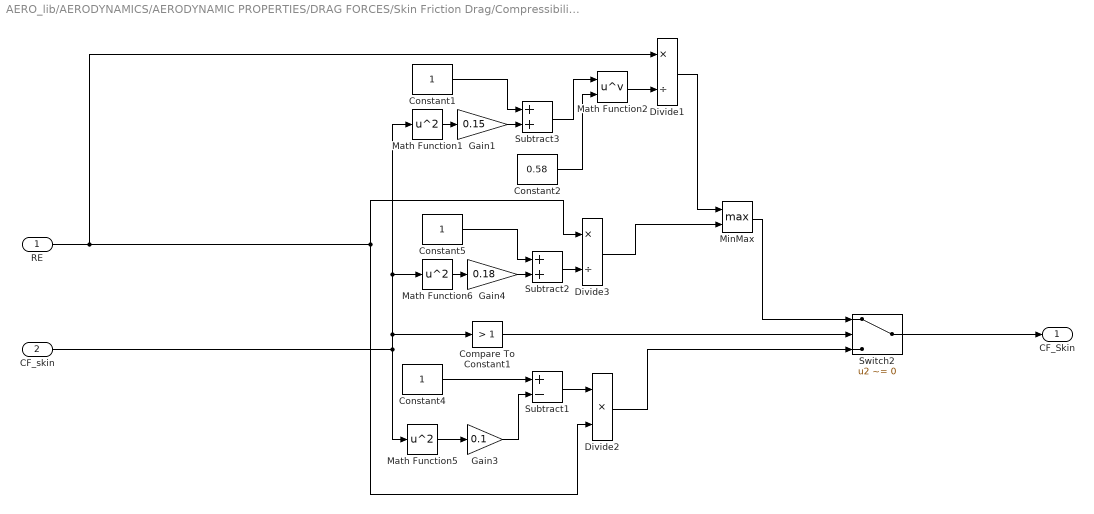
== system AERO_lib/AERODYNAMICS/AERODYNAMIC PROPERTIES/DRAG FORCES/Skin Friction Drag/Compressibility Corrections ==
  RE : Inport
  CF_skin : Inport  Port=2
  Compare To Constant1 : simulink/Logic and Bit Operations/Compare To Constant  relop=>  const=1  OutDataTypeStr=boolean
  Constant1 : Constant
  Constant2 : Constant  Value=0.58
  Constant4 : Constant
  Constant5 : Constant
  Divide1 : Product  Inputs=*/
  Divide2 : Product  Inputs=**
  Divide3 : Product  Inputs=*/
  Gain1 : Gain  Gain=0.15
  Gain3 : Gain  Gain=0.1
  Gain4 : Gain  Gain=0.18
  Math Function1 : Math  Operator=square  SaturateOnIntegerOverflow=on
  Math Function2 : Math  Operator=pow  SaturateOnIntegerOverflow=on
  Math Function5 : Math  Operator=square  SaturateOnIntegerOverflow=on
  Math Function6 : Math  Operator=square  SaturateOnIntegerOverflow=on
  MinMax : MinMax  Function=max  Inputs=2
  Subtract1 : Sum  Inputs=+-
  Subtract2 : Sum
  Subtract3 : Sum
  Switch2 : Switch  Criteria=u2 ~= 0
  CF_Skin : Outport
  wires:
  Subtract1/1 -> Divide2/1
  Math Function2/1 -> Divide1/2
  Constant2/1 -> Math Function2/2
  Subtract3/1 -> Math Function2/1
  Math Function5/1 -> Gain3/1
  Gain3/1 -> Subtract1/2
  Constant4/1 -> Subtract1/1
  Divide2/1 -> Switch2/3
  Compare To Constant1/1 -> Switch2/2
  CF_skin/1 -> Math Function5/1, Math Function1/1, Math Function6/1, Compare To Constant1/1
  Constant1/1 -> Subtract3/1
  Gain1/1 -> Subtract3/2
  Math Function1/1 -> Gain1/1
  Math Function6/1 -> Gain4/1
  Gain4/1 -> Subtract2/2
  MinMax/1 -> Switch2/1
  RE/1 -> Divide1/1, Divide2/2, Divide3/1
  Subtract2/1 -> Divide3/2
  Divide3/1 -> MinMax/2
  Switch2/1 -> CF_Skin/1
  Constant5/1 -> Subtract2/1
  Divide1/1 -> MinMax/1

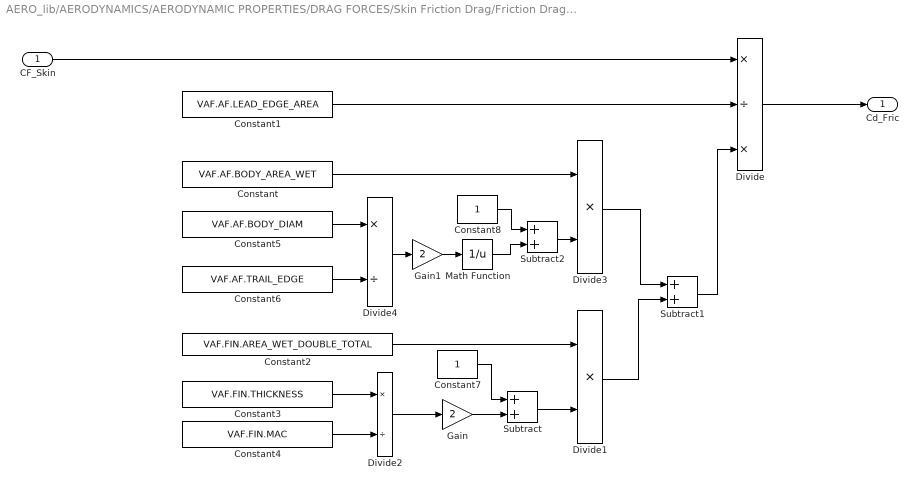
== system AERO_lib/AERODYNAMICS/AERODYNAMIC PROPERTIES/DRAG FORCES/Skin Friction Drag/Friction Drag Coefficient ==
  CF_Skin : Inport
  Constant : Constant  Value=VAF.AF.BODY_AREA_WET
  Constant1 : Constant  Value=VAF.AF.LEAD_EDGE_AREA
  Constant2 : Constant  Value=VAF.FIN.AREA_WET_DOUBLE_TOTAL
  Constant3 : Constant  Value=VAF.FIN.THICKNESS
  Constant4 : Constant  Value=VAF.FIN.MAC
  Constant5 : Constant  Value=VAF.AF.BODY_DIAM
  Constant6 : Constant  Value=VAF.AF.TRAIL_EDGE
  Constant7 : Constant
  Constant8 : Constant
  Divide : Product  Inputs=*/*
  Divide1 : Product  Inputs=**
  Divide2 : Product  Inputs=*/
  Divide3 : Product  Inputs=**
  Divide4 : Product  Inputs=*/
  Gain : Gain  Gain=2
  Gain1 : Gain  Gain=2
  Math Function : Math  Operator=reciprocal  SaturateOnIntegerOverflow=on
  Subtract : Sum
  Subtract1 : Sum
  Subtract2 : Sum
  Cd_Fric : Outport
  wires:
  Gain1/1 -> Math Function/1
  Divide/1 -> Cd_Fric/1
  Divide4/1 -> Gain1/1
  Gain/1 -> Subtract/2
  Constant7/1 -> Subtract/1
  Constant/1 -> Divide3/1
  CF_Skin/1 -> Divide/1
  Subtract2/1 -> Divide3/2
  Constant8/1 -> Subtract2/1
  Math Function/1 -> Subtract2/2
  Subtract1/1 -> Divide/3
  Divide1/1 -> Subtract1/2
  Divide3/1 -> Subtract1/1
  Constant2/1 -> Divide1/1
  Constant6/1 -> Divide4/2
  Constant5/1 -> Divide4/1
  Divide2/1 -> Gain/1
  Constant1/1 -> Divide/2
  Subtract/1 -> Divide1/2
  Constant4/1 -> Divide2/2
  Constant3/1 -> Divide2/1

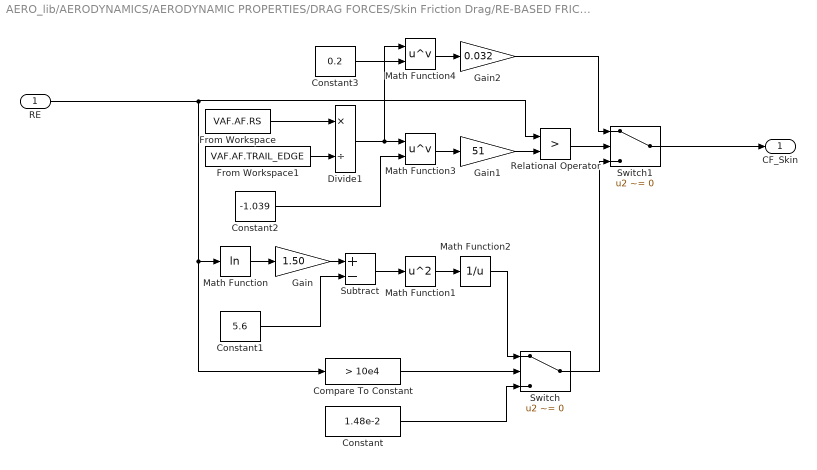
== system AERO_lib/AERODYNAMICS/AERODYNAMIC PROPERTIES/DRAG FORCES/Skin Friction Drag/RE-BASED FRIC. COEFF ==
  RE : Inport
  Compare To Constant : simulink/Logic and Bit Operations/Compare To Constant  relop=>  const=10e4  OutDataTypeStr=boolean
  Constant : Constant  Value=1.48e-2
  Constant1 : Constant  Value=5.6
  Constant2 : Constant  Value=-1.039
  Constant3 : Constant  Value=0.2
  Divide1 : Product  Inputs=*/
  From Workspace : FromWorkspace  VariableName=VAF.AF.RS  SampleTime=0
  From Workspace1 : FromWorkspace  VariableName=VAF.AF.TRAIL_EDGE  SampleTime=0
  Gain : Gain  Gain=1.50
  Gain1 : Gain  Gain=51
  Gain2 : Gain  Gain=0.032
  Math Function : Math  Operator=log  SaturateOnIntegerOverflow=on
  Math Function1 : Math  Operator=square  SaturateOnIntegerOverflow=on
  Math Function2 : Math  Operator=reciprocal  SaturateOnIntegerOverflow=on
  Math Function3 : Math  Operator=pow  SaturateOnIntegerOverflow=on
  Math Function4 : Math  Operator=pow  SaturateOnIntegerOverflow=on
  Relational Operator : RelationalOperator  Operator=>  OutDataTypeStr=boolean
  Subtract : Sum  Inputs=+-
  Switch : Switch  Criteria=u2 ~= 0
  Switch1 : Switch  Criteria=u2 ~= 0
  CF_Skin : Outport
  wires:
  Switch1/1 -> CF_Skin/1
  Compare To Constant/1 -> Switch/2
  From Workspace/1 -> Divide1/1
  From Workspace1/1 -> Divide1/2
  Subtract/1 -> Math Function1/1
  Math Function2/1 -> Switch/1
  Math Function1/1 -> Math Function2/1
  Constant3/1 -> Math Function4/2
  Math Function4/1 -> Gain2/1
  Gain2/1 -> Switch1/1
  Math Function/1 -> Gain/1
  Switch/1 -> Switch1/3
  Constant/1 -> Switch/3
  Relational Operator/1 -> Switch1/2
  Gain1/1 -> Relational Operator/2
  Constant2/1 -> Math Function3/2
  Divide1/1 -> Math Function4/1, Math Function3/1
  Math Function3/1 -> Gain1/1
  RE/1 -> Math Function/1, Compare To Constant/1, Relational Operator/1
  Constant1/1 -> Subtract/2
  Gain/1 -> Subtract/1

== system AERO_lib/AERODYNAMICS/AERODYNAMIC PROPERTIES/Center of Pressure/FIN_CP/FIN CP/CP_SUPERSONIC ==
  Mach : Inport
  ASPECT RATIO : FromWorkspace  VariableName=VAF.FIN.ASPECT_RATIO
  Constant : Constant
  Constant1 : Constant  Value=0.67
  Constant2 : Constant
  Divide : Product  Inputs=**/
  Gain : Gain  Gain=2
  MAC : FromWorkspace  VariableName=VAF.FIN.MAC
  Math Function : Math  Operator=square  SaturateOnIntegerOverflow=on
  Product : Product
  Sqrt : Sqrt  SaturateOnIntegerOverflow=on
  Subtract : Sum  Inputs=+-
  Subtract1 : Sum  Inputs=+-
  Subtract2 : Sum  Inputs=+-
  X_F_SUPERSONIC : Outport
  wires:
  Mach/1 -> Math Function/1
  Constant/1 -> Subtract/2
  Math Function/1 -> Subtract/1
  Subtract/1 -> Sqrt/1
  Sqrt/1 -> Product/1
  ASPECT RATIO/1 -> Product/2
  Product/1 -> Gain/1, Subtract1/1
  Constant1/1 -> Subtract1/2
  Constant2/1 -> Subtract2/2
  Subtract1/1 -> Divide/2
  Subtract2/1 -> Divide/3
  Divide/1 -> X_F_SUPERSONIC/1
  Gain/1 -> Subtract2/1
  MAC/1 -> Divide/1

== system AERO_lib/AERODYNAMICS/AERODYNAMIC PROPERTIES/Center of Pressure/FIN_CP/SINGLE FIN CN_ALPHA/BETA ==
  MACH : Inport
  Compare To Constant2 : simulink/Logic and Bit Operations/Compare To Constant  relop=>  const=1  OutDataTypeStr=boolean
  Constant : Constant
  Constant1 : Constant
  Math Function : Math  Operator=square  SaturateOnIntegerOverflow=on
  Math Function1 : Math  Operator=square  SaturateOnIntegerOverflow=on
  Sqrt : Sqrt  SaturateOnIntegerOverflow=on
  Subtract : Sum  Inputs=+-
  Subtract1 : Sum  Inputs=-+
  Switch3 : Switch  Criteria=u2 ~= 0
  BETA : Outport
  wires:
  Switch3/1 -> Sqrt/1
  Subtract1/1 -> Switch3/3
  Constant1/1 -> Subtract1/2
  Math Function1/1 -> Subtract1/1
  Constant/1 -> Subtract/2
  Subtract/1 -> Switch3/1
  Math Function/1 -> Subtract/1
  MACH/1 -> Math Function/1, Math Function1/1, Compare To Constant2/1
  Sqrt/1 -> BETA/1
  Compare To Constant2/1 -> Switch3/2

== system AERO_lib/AERODYNAMICS/AERODYNAMIC PROPERTIES/DRAG FORCES/Body Drag/BASE/Subsonic ==
  note: CD_LE = 1 + M^2/4 + M^4 / 40
  MACH : Inport
  Action Port : ActionPort
  Constant : Constant  Value=0.12
  Gain : Gain  Gain=0.13
  Math Function : Math  Operator=square  SaturateOnIntegerOverflow=on
  Subtract : Sum
  CD_BASE : Outport
  wires:
  Constant/1 -> Subtract/2
  Math Function/1 -> Gain/1
  MACH/1 -> Math Function/1
  Subtract/1 -> CD_BASE/1
  Gain/1 -> Subtract/1

== system AERO_lib/AERODYNAMICS/AERODYNAMIC PROPERTIES/DRAG FORCES/Body Drag/BASE/Supersonic ==
  MACH : Inport
  Action Port : ActionPort
  Gain : Gain  Gain=0.25
  Math Function : Math  Operator=reciprocal  SaturateOnIntegerOverflow=on
  CD_BASE : Outport
  wires:
  Gain/1 -> CD_BASE/1
  MACH/1 -> Math Function/1
  Math Function/1 -> Gain/1

== system AERO_lib/AERODYNAMICS/AERODYNAMIC PROPERTIES/DRAG FORCES/Body Drag/FINS/Leading Edge ==
  MACH : Inport
  Constant : Constant  Value=VAF.FIN.ROUNDED_LEADING_EDGE
  Constant1 : Constant  Value=VAF.FIN.SWEEP
  Constant2 : Constant  Value=VAF.FIN.SPAN
  Divide : Product  Inputs=**
  Divide1 : Product  Inputs=*/
  Rectangular Leading Edge : Subsystem
  Rounded Leading Edge : Subsystem
  Switch : Switch  Criteria=u2 ~= 0
  Trigonometric Function : Trigonometry  Operator=atan
  CD_FIN_LE : Outport
  wires:
  Rounded Leading Edge/1(CD_FIN_LE) -> Switch/1
  Rectangular Leading Edge/1(CD_FIN_LE) -> Switch/3
  Constant/1 -> Switch/2
  Constant2/1 -> Divide1/2
  Constant1/1 -> Divide1/1
  Switch/1 -> Divide/1
  Trigonometric Function/1 -> Divide/2
  Divide1/1 -> Trigonometric Function/1
  MACH/1 -> Rounded Leading Edge/1(MACH), Rectangular Leading Edge/1(MACH)
  Divide/1 -> CD_FIN_LE/1

== system AERO_lib/AERODYNAMICS/AERODYNAMIC PROPERTIES/DRAG FORCES/Body Drag/FINS/Trailing Edge ==
  MACH : Inport
  Add1 : Sum
  Constant : Constant  Value=VAF.ROUND_TRAIL_EDGE
  Constant1 : Constant  Value=VAF.TAPER_TRAIL_EDGE
  Constant2 : Constant  Value=0
  Gain : Gain  Gain=0.5
  If : If  IfExpression=u1<1
  Subsonic : Subsystem  TreatAsAtomicUnit=on
  Supersonic : Subsystem  TreatAsAtomicUnit=on
  Switch : Switch  Criteria=u2 ~= 0
  Switch1 : Switch  Criteria=u2 ~= 0
  CD_FIN_LE : Outport
  wires:
  If/2 -> Supersonic/Action
  If/1 -> Subsonic/Action
  Subsonic/1(CD_FIN_LE) -> Add1/2
  Supersonic/1(CD_FIN_LE) -> Add1/1
  MACH/1 -> Supersonic/1(MACH), Subsonic/1(MACH), If/1
  Add1/1 -> Gain/1, Switch/3
  Constant/1 -> Switch/2
  Gain/1 -> Switch/1
  Switch/1 -> Switch1/3
  Switch1/1 -> CD_FIN_LE/1
  Constant1/1 -> Switch1/2
  Constant2/1 -> Switch1/1

== system AERO_lib/AERODYNAMICS/AERODYNAMIC PROPERTIES/DRAG FORCES/Body Drag/NOSE/HIGH SUBSONIC ==
  MACH : Inport
  Action Port : ActionPort
  Add : Sum
  Add1 : Sum  Inputs=-+
  Divide : Product  Inputs=**
  Gain : Gain  Gain=4/2.4
  Low Subsonic Cd : Constant  Value=VAF.NC.CD_PRESSURE_SUBSONIC;
  Math Function : Math  Operator=pow  SaturateOnIntegerOverflow=on
  Math Function1 : Math  Operator=reciprocal  SaturateOnIntegerOverflow=on
  Transonic Cd : Constant  Value=VAF.NC.CD_TRANSONIC
  Transonic Cd1 : Constant  Value=0.5
  Cd_NC : Outport
  wires:
  Add/1 -> Cd_NC/1
  Divide/1 -> Add/1
  MACH/1 -> Math Function/1
  Math Function/1 -> Divide/1
  Low Subsonic Cd/1 -> Add/2
  Transonic Cd/1 -> Math Function1/1, Divide/2
  Math Function1/1 -> Add1/2
  Transonic Cd1/1 -> Add1/1
  Add1/1 -> Gain/1
  Gain/1 -> Math Function/2

== system AERO_lib/AERODYNAMICS/AERODYNAMIC PROPERTIES/DRAG FORCES/Body Drag/NOSE/LOW SUBSONIC ==
  Action Port : ActionPort
  Constant : Constant  Value=VAF.NC.CD_PRESSURE_SUBSONIC
  Out1 : Outport
  wires:
  Constant/1 -> Out1/1

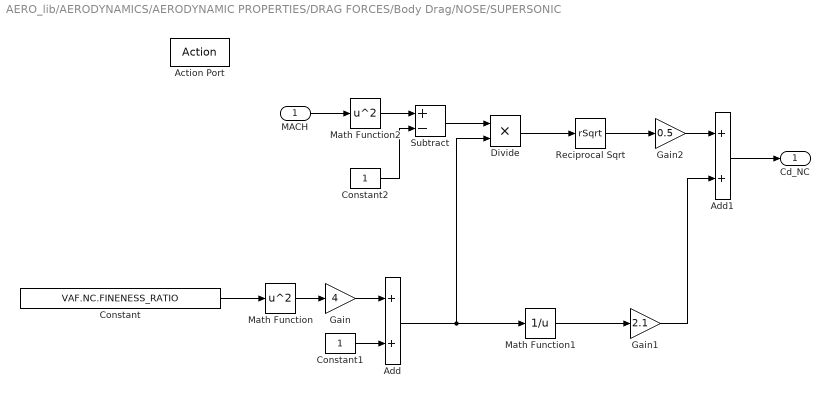
== system AERO_lib/AERODYNAMICS/AERODYNAMIC PROPERTIES/DRAG FORCES/Body Drag/NOSE/SUPERSONIC ==
  MACH : Inport
  Action Port : ActionPort
  Add : Sum
  Add1 : Sum
  Constant : Constant  Value=VAF.NC.FINENESS_RATIO
  Constant1 : Constant
  Constant2 : Constant
  Divide : Product  Inputs=**
  Gain : Gain  Gain=4
  Gain1 : Gain  Gain=2.1
  Gain2 : Gain  Gain=0.5
  Math Function : Math  Operator=square  SaturateOnIntegerOverflow=on
  Math Function1 : Math  Operator=reciprocal  SaturateOnIntegerOverflow=on
  Math Function2 : Math  Operator=square  SaturateOnIntegerOverflow=on
  Reciprocal Sqrt : Sqrt  Operator=rSqrt  SaturateOnIntegerOverflow=on
  Subtract : Sum  Inputs=+-
  Cd_NC : Outport
  wires:
  Constant/1 -> Math Function/1
  Math Function/1 -> Gain/1
  Gain/1 -> Add/1
  Constant1/1 -> Add/2
  Add1/1 -> Cd_NC/1
  Gain1/1 -> Add1/2
  Math Function1/1 -> Gain1/1
  Add/1 -> Divide/2, Math Function1/1
  Gain2/1 -> Add1/1
  Reciprocal Sqrt/1 -> Gain2/1
  Divide/1 -> Reciprocal Sqrt/1
  Subtract/1 -> Divide/1
  MACH/1 -> Math Function2/1
  Math Function2/1 -> Subtract/1
  Constant2/1 -> Subtract/2

== system AERO_lib/AERODYNAMICS/AERODYNAMIC PROPERTIES/DRAG FORCES/Body Drag/NOSE/TRANSONIC ==
  MACH : Inport
  Action Port : ActionPort
  Constant : Constant  Value=VAF.NC.TRASONIC_CONSTANTS
  Constant1 : Constant
  Dot Product : DotProduct  InputSameDT=on  OutDataTypeStr=Inherit: Inherit via internal rule
  Math Function : Math  Operator=square  SaturateOnIntegerOverflow=on
  Mux : Mux  Inputs=3
  Cd_NC : Outport
  wires:
  MACH/1 -> Mux/2, Math Function/1
  Constant1/1 -> Mux/3
  Mux/1 -> Dot Product/1
  Constant/1 -> Dot Product/2
  Math Function/1 -> Mux/1
  Dot Product/1 -> Cd_NC/1

== system AERO_lib/AERODYNAMICS/AERODYNAMIC PROPERTIES/DRAG FORCES/Body Drag/PARASITIC/CD_STAG ==
  MACH : Inport
  Add1 : Sum
  If : If  IfExpression=u1<1
  Subsonic : Subsystem  TreatAsAtomicUnit=on
  Supersonic : Subsystem  TreatAsAtomicUnit=on
  CD_STAG : Outport
  wires:
  MACH/1 -> If/1, Subsonic/1(MACH), Supersonic/1(MACH)
  Supersonic/1(CD_STAG) -> Add1/1
  Subsonic/1(CD_STAG) -> Add1/2
  If/1 -> Subsonic/Action
  If/2 -> Supersonic/Action
  Add1/1 -> CD_STAG/1

== system AERO_lib/AERODYNAMICS/AERODYNAMIC PROPERTIES/DRAG FORCES/Body Drag/FINS/Leading Edge/Rectangular Leading Edge ==
  MACH : Inport
  Add1 : Sum
  If : If  IfExpression=u1<1
  Subsonic : Subsystem  TreatAsAtomicUnit=on
  Supersonic : Subsystem  TreatAsAtomicUnit=on
  CD_FIN_LE : Outport
  wires:
  MACH/1 -> If/1, Subsonic/1(MACH), Supersonic/1(MACH)
  Supersonic/1(CD_FIN_LE) -> Add1/1
  Subsonic/1(CD_FIN_LE) -> Add1/2
  If/1 -> Subsonic/Action
  If/2 -> Supersonic/Action
  Add1/1 -> CD_FIN_LE/1

== system AERO_lib/AERODYNAMICS/AERODYNAMIC PROPERTIES/DRAG FORCES/Body Drag/FINS/Leading Edge/Rounded Leading Edge ==
  MACH : Inport
  Add1 : Sum  Inputs=+++
  If : If  IfExpression=u1<0.9  ElseIfExpressions=u1>1
  Subsonic : Subsystem  TreatAsAtomicUnit=on
  Supersonic : Subsystem  TreatAsAtomicUnit=on
  Transonic : Subsystem  TreatAsAtomicUnit=on
  CD_FIN_LE : Outport
  wires:
  Add1/1 -> CD_FIN_LE/1
  If/3 -> Transonic/Action
  If/1 -> Subsonic/Action
  If/2 -> Supersonic/Action
  Subsonic/1(CD_FIN_LE) -> Add1/3
  Transonic/1(CD_FIN_LE) -> Add1/1
  Supersonic/1(CD_FIN_LE) -> Add1/2
  MACH/1 -> Transonic/1(MACH), Supersonic/1(MACH), Subsonic/1(MACH), If/1

== system AERO_lib/AERODYNAMICS/AERODYNAMIC PROPERTIES/DRAG FORCES/Body Drag/FINS/Trailing Edge/Subsonic ==
  note: CD_LE = 1 + M^2/4 + M^4 / 40
  MACH : Inport
  Action Port : ActionPort
  Constant : Constant  Value=0.12
  Gain : Gain  Gain=0.13
  Math Function : Math  Operator=square  SaturateOnIntegerOverflow=on
  Subtract : Sum
  CD_FIN_LE : Outport
  wires:
  Gain/1 -> Subtract/1
  Subtract/1 -> CD_FIN_LE/1
  MACH/1 -> Math Function/1
  Math Function/1 -> Gain/1
  Constant/1 -> Subtract/2

== system AERO_lib/AERODYNAMICS/AERODYNAMIC PROPERTIES/DRAG FORCES/Body Drag/FINS/Trailing Edge/Supersonic ==
  MACH : Inport
  Action Port : ActionPort
  Gain : Gain  Gain=0.25
  Math Function : Math  Operator=reciprocal  SaturateOnIntegerOverflow=on
  CD_FIN_LE : Outport
  wires:
  Math Function/1 -> Gain/1
  MACH/1 -> Math Function/1
  Gain/1 -> CD_FIN_LE/1

== system AERO_lib/AERODYNAMICS/AERODYNAMIC PROPERTIES/DRAG FORCES/Body Drag/PARASITIC/CD_STAG/Subsonic ==
  note: CD_LE = 1 + M^2/4 + M^4 / 40
  MACH : Inport
  Action Port : ActionPort
  Constant : Constant
  Gain : Gain  Gain=0.25
  Gain1 : Gain  Gain=1/40
  Math Function : Math  Operator=square  SaturateOnIntegerOverflow=on
  Math Function1 : Math  Operator=square  SaturateOnIntegerOverflow=on
  Subtract : Sum  Inputs=+++
  CD_STAG : Outport
  wires:
  Math Function/1 -> Gain/1, Math Function1/1
  MACH/1 -> Math Function/1
  Subtract/1 -> CD_STAG/1
  Gain/1 -> Subtract/1
  Math Function1/1 -> Gain1/1
  Gain1/1 -> Subtract/2
  Constant/1 -> Subtract/3

== system AERO_lib/AERODYNAMICS/AERODYNAMIC PROPERTIES/DRAG FORCES/Body Drag/PARASITIC/CD_STAG/Supersonic ==
  MACH : Inport
  Action Port : ActionPort
  Add : Sum  Inputs=+-++
  Constant : Constant  Value=1.84
  Gain : Gain  Gain=0.76
  Gain1 : Gain  Gain=0.166
  Gain2 : Gain  Gain=0.035
  Math Function : Math  Operator=reciprocal  SaturateOnIntegerOverflow=on
  Math Function1 : Math  Operator=square  SaturateOnIntegerOverflow=on
  Math Function2 : Math  Operator=square  SaturateOnIntegerOverflow=on
  Product : Product
  CD_STAG : Outport
  wires:
  Gain/1 -> Add/2
  Constant/1 -> Add/1
  Add/1 -> CD_STAG/1
  MACH/1 -> Math Function/1
  Math Function/1 -> Math Function1/1
  Math Function2/1 -> Gain1/1, Product/1
  Math Function1/1 -> Math Function2/1, Product/2, Gain/1
  Product/1 -> Gain2/1
  Gain1/1 -> Add/3
  Gain2/1 -> Add/4

== system AERO_lib/AERODYNAMICS/AERODYNAMIC PROPERTIES/DRAG FORCES/Body Drag/FINS/Leading Edge/Rectangular Leading Edge/Subsonic ==
  note: CD_LE = 1 + M^2/4 + M^4 / 40
  MACH : Inport
  Action Port : ActionPort
  Constant : Constant
  Gain : Gain  Gain=0.25
  Gain1 : Gain  Gain=1/40
  Math Function : Math  Operator=square  SaturateOnIntegerOverflow=on
  Math Function1 : Math  Operator=square  SaturateOnIntegerOverflow=on
  Subtract : Sum  Inputs=+++
  CD_FIN_LE : Outport
  wires:
  Math Function/1 -> Gain/1, Math Function1/1
  MACH/1 -> Math Function/1
  Subtract/1 -> CD_FIN_LE/1
  Gain/1 -> Subtract/1
  Math Function1/1 -> Gain1/1
  Gain1/1 -> Subtract/2
  Constant/1 -> Subtract/3

== system AERO_lib/AERODYNAMICS/AERODYNAMIC PROPERTIES/DRAG FORCES/Body Drag/FINS/Leading Edge/Rectangular Leading Edge/Supersonic ==
  MACH : Inport
  Action Port : ActionPort
  Add : Sum  Inputs=+-++
  Constant : Constant  Value=1.84
  Gain : Gain  Gain=0.76
  Gain1 : Gain  Gain=0.166
  Gain2 : Gain  Gain=0.035
  Math Function : Math  Operator=reciprocal  SaturateOnIntegerOverflow=on
  Math Function1 : Math  Operator=square  SaturateOnIntegerOverflow=on
  Math Function2 : Math  Operator=square  SaturateOnIntegerOverflow=on
  Product : Product
  CD_FIN_LE : Outport
  wires:
  Gain/1 -> Add/2
  Constant/1 -> Add/1
  Add/1 -> CD_FIN_LE/1
  MACH/1 -> Math Function/1
  Math Function/1 -> Math Function1/1
  Math Function2/1 -> Gain1/1, Product/1
  Math Function1/1 -> Math Function2/1, Product/2, Gain/1
  Product/1 -> Gain2/1
  Gain1/1 -> Add/3
  Gain2/1 -> Add/4

== system AERO_lib/AERODYNAMICS/AERODYNAMIC PROPERTIES/DRAG FORCES/Body Drag/FINS/Leading Edge/Rounded Leading Edge/Subsonic ==
  note: CD_LE = (1 - M^2) ^(-0.417) - 1
  MACH : Inport
  Action Port : ActionPort
  Constant : Constant
  Constant1 : Constant  Value=-0.417
  Constant2 : Constant
  Math Function : Math  Operator=square  SaturateOnIntegerOverflow=on
  Math Function1 : Math  Operator=pow  SaturateOnIntegerOverflow=on
  Subtract : Sum  Inputs=+-
  Subtract1 : Sum  Inputs=+-
  CD_FIN_LE : Outport
  wires:
  MACH/1 -> Math Function/1
  Math Function/1 -> Subtract/1
  Constant/1 -> Subtract/2
  Subtract/1 -> Math Function1/1
  Constant1/1 -> Math Function1/2
  Math Function1/1 -> Subtract1/1
  Constant2/1 -> Subtract1/2
  Subtract1/1 -> CD_FIN_LE/1

== system AERO_lib/AERODYNAMICS/AERODYNAMIC PROPERTIES/DRAG FORCES/Body Drag/FINS/Leading Edge/Rounded Leading Edge/Supersonic ==
  MACH : Inport
  Action Port : ActionPort
  Add : Sum  Inputs=+-+
  Constant1 : Constant  Value=1.214
  Constant2 : Constant  Value=4
  Gain : Gain  Gain=0.502
  Gain1 : Gain  Gain=0.1095
  Math Function : Math  Operator=pow  SaturateOnIntegerOverflow=on
  Math Function1 : Math  Operator=square  SaturateOnIntegerOverflow=on
  Math Function2 : Math  Operator=reciprocal  SaturateOnIntegerOverflow=on
  CD_FIN_LE : Outport
  wires:
  Constant1/1 -> Add/3
  MACH/1 -> Math Function2/1
  Math Function2/1 -> Math Function1/1, Math Function/1
  Math Function1/1 -> Gain/1
  Gain/1 -> Add/2
  Constant2/1 -> Math Function/2
  Add/1 -> CD_FIN_LE/1
  Math Function/1 -> Gain1/1
  Gain1/1 -> Add/1

== system AERO_lib/AERODYNAMICS/AERODYNAMIC PROPERTIES/DRAG FORCES/Body Drag/FINS/Leading Edge/Rounded Leading Edge/Transonic ==
  MACH : Inport
  Action Port : ActionPort
  Add : Sum  Inputs=-+
  Add1 : Sum  Inputs=+-
  Constant : Constant
  Constant1 : Constant  Value=0.9
  Gain : Gain  Gain=1.785
  CD_FIN_LE : Outport
  wires:
  Add/1 -> CD_FIN_LE/1
  Constant/1 -> Add/1
  MACH/1 -> Add1/1
  Constant1/1 -> Add1/2
  Add1/1 -> Gain/1
  Gain/1 -> Add/2
